simulink model "R4"  (R2018a)
settings: Solver=VariableStepAuto  StartTime=0.0  StopTime=10.0  RelTol=1e-3
undefined symbols (not defined in the file): k
libraries: commdigbbndfm2 x2, commchan3 x1, commsink2 x1, commrandsrc3 x1
settings Model: Creator=Prof. S.R.Singh  LastModifiedBy=Prof. S.R.Singh

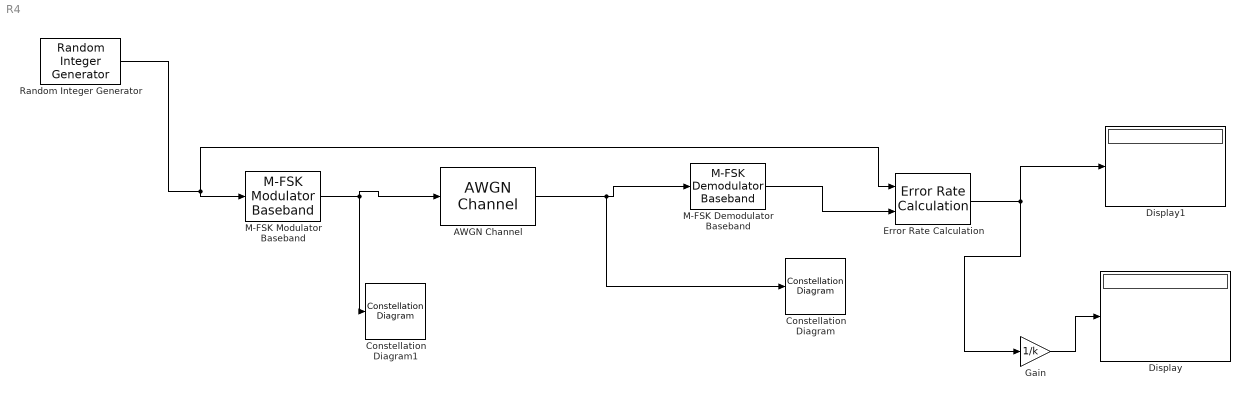
== system R4 ==
  AWGN Channel : commchan3/AWGN Channel  InputProcessing=Columns as channels (frame based)  seed=67  noiseMode="Signal to noise ratio  (Eb/No)"  EbNodB=5 + 10*log10(k)  EsNodB=10  SNRdB=10  bitsPerSym=1  Ps=1  Tsym=1  variance=1
  Constellation Diagram : ConstellationDiagram
  Constellation Diagram1 : ConstellationDiagram
  Display : Display
  Display1 : Display
      settings: Decimation=3
  Error Rate Calculation : commsink2/Error Rate Calculation  N=0  st_delay=0  cp_mode=Entire frame  subframe=[]  PMode=Port  WsName=ErrorVec  RsMode2=off  stop=off  numErr=100  maxBits=1e6
  Gain : Gain  Gain=1/k
  M-FSK Demodulator Baseband : commdigbbndfm2/M-FSK Demodulator Baseband  M=M  OutType=Integer  Dec=Gray  freqSep=6  numSamp=17  RateOptions=Enforce single-rate processing  outDataType=double
      settings: SourceProductName=Communications System Toolbox  SourceProductBaseCode=CM
  M-FSK Modulator Baseband : commdigbbndfm2/M-FSK Modulator Baseband  M=M  InType=Integer  Enc=Gray  freqSep=6  phaseType=Continuous  numSamp=17  RateOptions=Enforce single-rate processing  outDataType=double
      settings: SourceProductName=Communications System Toolbox
  Random Integer Generator : commrandsrc3/Random Integer Generator  SetSize=M  SeedSource=Auto  Seed=0  SampleTime=1  SamplesPerFrame=1  OutputDataType=double  SimulateUsing=Interpreted execution
  wires:
  M-FSK Modulator Baseband/1 -> AWGN Channel/1, Constellation Diagram1/1
  Random Integer Generator/1 -> M-FSK Modulator Baseband/1, Error Rate Calculation/1
  Error Rate Calculation/1 -> Display1/1, Gain/1
  Gain/1 -> Display/1
  AWGN Channel/1 -> M-FSK Demodulator Baseband/1, Constellation Diagram/1
  M-FSK Demodulator Baseband/1 -> Error Rate Calculation/2
